simulink model "Einfachpendel_mit_Agent_19_09_22_17_13_35"  (R2022a)
settings: Solver=VariableStepAuto  StartTime=0.0  StopTime=Tf  RelTol=1e-3
PreLoadFcn:
  | init_Einfachpendel_mit_Agent
undefined symbols (not defined in the file or in its folder): d, Sample, theta0, X, x_lim, x_tar, Y, Z
libraries: sm_lib x15, nesl_utility x7, simulink x1, rllib x1
settings Model: Creator=ELSYS-PC3  LastModifiedBy=ts
settings SolverCC: AlgebraicLoopSolver=TrustRegion
settings DebuggingCC: UnconnectedInputMsg=warning  UnconnectedOutputMsg=warning  UnconnectedLineMsg=warning  SFMachineParentedDataDiag=warning  ArithmeticOperatorsInVariantConditions=warning
settings SFSimCC: SimUseLocalCustomCode=off  CustomCodeUndefinedFunction=UseInterfaceOnly
settings RTWCC: RTWUseLocalCustomCode=off  DLArmComputeVersion=19.05

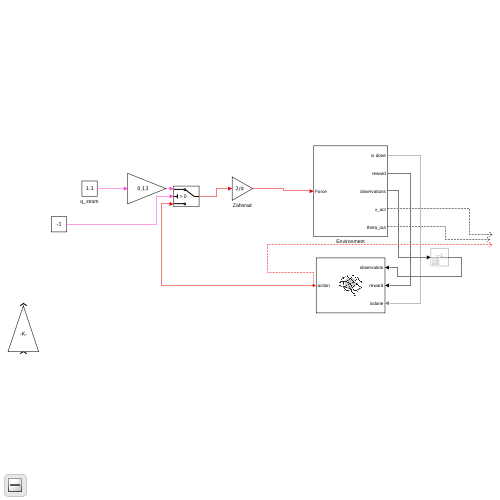
[thumbnail: Simulink's stored preview of the top-level diagram]
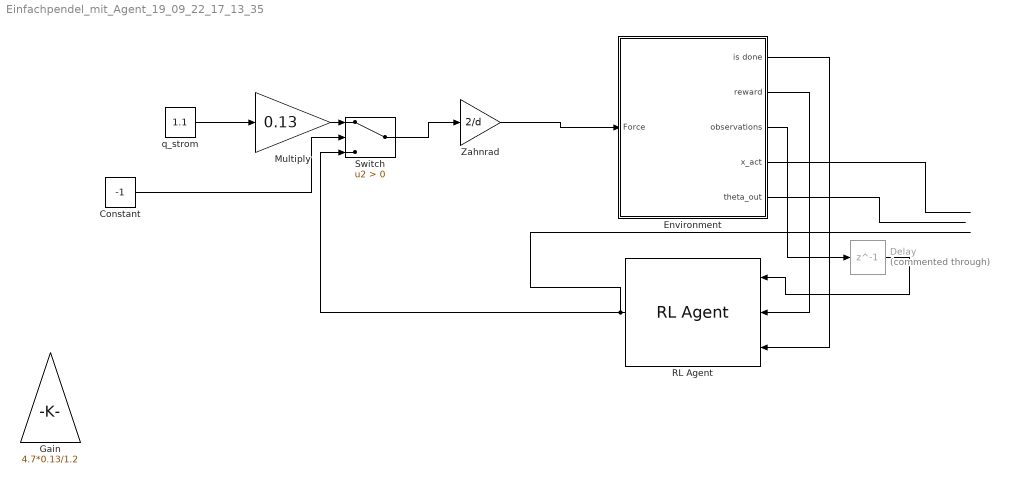
== system Einfachpendel_mit_Agent_19_09_22_17_13_35 ==
  Constant : Constant  Value=-1
  Delay : Delay  Commented=through  DelayLength=1
  Environment : Subsystem
  Gain : Gain  Gain=4.7*0.13/1.2
  Multiply : Gain  Gain=0.13
  RL Agent : rllib/RL Agent  Agent=bestagent  ExternalActionAsInput=off  ProvideLastAction=off  ProvideCumRwd=off  TreatAsDirectFeedthrough=on  UseStrictObservationDataTypes=off
  Switch : Switch  Criteria=u2 > Threshold  SaturateOnIntegerOverflow=off  InputSameDT=off
  Zahnrad : Gain  Gain=2/d
  q_strom : Constant  Value=1.1
  wires:
  Environment/1(is done) -> RL Agent/3
  Environment/2(reward) -> RL Agent/2
  Environment/4(x_act) -> ?
  Environment/5(theta_out) -> ?
  Environment/3(observations) -> Delay/1
  Delay/1 -> RL Agent/1
  Zahnrad/1 -> Environment/1(Force)
  q_strom/1 -> Multiply/1
  Switch/1 -> Zahnrad/1
  Constant/1 -> Switch/2
  Multiply/1 -> Switch/1
  RL Agent/1 -> Switch/3

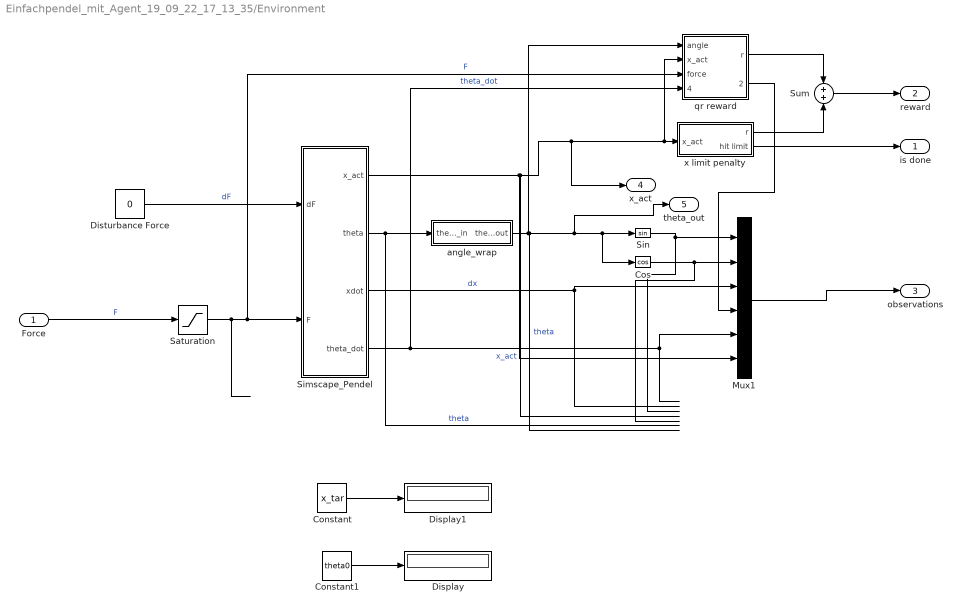
== system Einfachpendel_mit_Agent_19_09_22_17_13_35/Environment ==
  Force : Inport
  Constant : Constant  Value=x_tar
  Constant1 : Constant  Value=theta0
  Cos : Trigonometry  Operator=cos
  Display : Display
  Display1 : Display
  Disturbance Force : Constant  Value=0
  Mux1 : Mux  Inputs=6
  Saturation : Saturate  UpperLimit=140  LowerLimit=-140
  Simscape_Pendel : Subsystem
  Sin : Trigonometry
  Sum : Sum
  angle_wrap : Subsystem
  qr reward : Subsystem
  x limit penalty : Subsystem
  is done : Outport  VectorParamsAs1DForOutWhenUnconnected=off
  reward : Outport  Port=2  VectorParamsAs1DForOutWhenUnconnected=off
  observations : Outport  Port=3  VectorParamsAs1DForOutWhenUnconnected=off
  x_act : Outport  Port=4
  theta_out : Outport  Port=5
  wires:
  Mux1/1 -> observations/1
  Simscape_Pendel/3(xdot) -> Mux1/3  "dx"
  Simscape_Pendel/2("theta ") -> angle_wrap/1(theta_in)  "theta"
  Disturbance Force/1 -> Simscape_Pendel/1(dF)  "dF"
  angle_wrap/1(theta_out) -> theta_out/1, Cos/1, Sin/1, qr reward/1(angle)  "theta"
  Simscape_Pendel/4(theta_dot) -> qr reward/4(theta_dot), Mux1/5  "theta_dot"
  Sin/1 -> Mux1/1
  Cos/1 -> Mux1/2
  Sum/1 -> reward/1
  x limit penalty/2(hit limit) -> is done/1
  Saturation/1 -> Simscape_Pendel/2("F "), qr reward/3(force)  "F"
  qr reward/1(r) -> Sum/1
  x limit penalty/1(r) -> Sum/2
  Simscape_Pendel/1(x_act) -> Mux1/6, x_act/1, qr reward/2(x_act), x limit penalty/1(x_act)  "x_act"
  Force/1 -> Saturation/1  "F"
  Constant1/1 -> Display/1
  Constant/1 -> Display1/1
  qr reward/2(x_error) -> Mux1/4

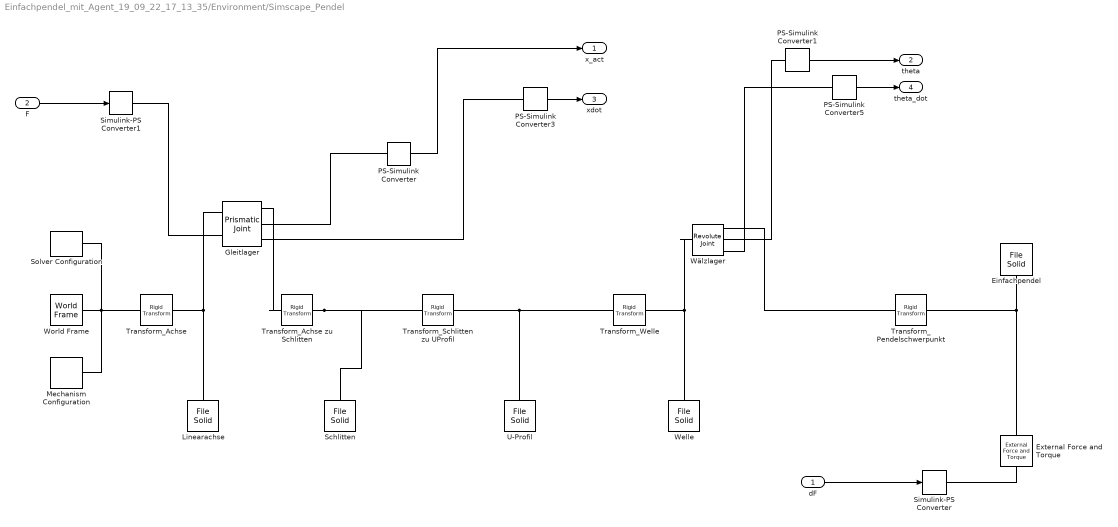
== system Einfachpendel_mit_Agent_19_09_22_17_13_35/Environment/Simscape_Pendel ==
  dF : Inport
  "F " : Inport  Port=2
  Einfachpendel : sm_lib/Body Elements/File Solid  ExtGeomFileName=/home/ts/Documents/2022_03_rosner_project2/Matlab/Pendel/V5_Einfachpendel_mit_Sollwertvorgabe/pendel2.stp  UnitType=FromFile  ExtGeomFileUnits=m  StepReaderType=OCC  ExportConvexHullGeometry=off  InertiaType=CalculateFromGeometry  Mass=1  MassUnits=kg  CenterOfMass=[0 0 0]  CenterOfMassUnits=m  MomentsOfInertia=[1 1 1]  MomentsOfInertiaUnits=kg*m^2  ProductsOfInertia=[0 0 0]  ProductsOfInertiaUnits=kg*m^2  BasedOnType=Density  Density=2710  DensityUnits=kg/m^3  DoExposeReferenceFrame=on  SerializedFrames=<Frames><Frame><Id>Frame1</Id><Value><Name>F1</Name><Origin><Source>CenterOfMassFrame</Source><FeatureName></FeatureName></Origin><PrimaryAxis><DefinedDirection>+Z</DefinedDirection><Source>ReferenceFrame</Source><SourceDirection>+Z</SourceDirection><FeatureName></FeatureName></PrimaryAxis><SecondaryAxis><DefinedDirection>+X</DefinedDirection><Source>ReferenceFrame</Source><SourceDirection>+X</SourceDirection><FeatureName></FeatureName></SecondaryAxis></Value></Frame></Frames>  GraphicType=FromGeometry  MarkerShape=Sphere  MarkerSize=10  GraphicVisPropType=SimpleVisualProperties  GraphicDiffuseColor=[1.0 0.2 0.4]  GraphicSpecularColor=[0.5 0.5 0.5 1.0]  GraphicAmbientColor=[0.15 0.15 0.15 1.0]  GraphicEmissiveColor=[0.0 0.0 0.0 1.0]  GraphicShininess=75  GraphicOpacity=1.0
  External Force and Torque : sm_lib/Forces and Torques/External Force and Torque  ForceResolutionFrame=AttachedFrame  EnableForceX=on  EnableForceY=off  EnableForceZ=off  EnableForce=off  TorqueResolutionFrame=AttachedFrame  EnableTorqueX=off  EnableTorqueY=off  EnableTorqueZ=off  EnableTorque=off
  Gleitlager : sm_lib/Joints/Prismatic Joint  JointMode=Normal  SenseConstraintForce=off  SenseConstraintForceX=off  SenseConstraintForceY=off  SenseConstraintForceZ=off  SenseConstraintTorque=off  SenseConstraintTorqueX=off  SenseConstraintTorqueY=off  SenseConstraintTorqueZ=off  SenseTotalForce=off  SenseTotalForceX=off  SenseTotalForceY=off  SenseTotalForceZ=off  SenseTotalTorque=off  SenseTotalTorqueX=off  SenseTotalTorqueY=off  SenseTotalTorqueZ=off  CompositeWrenchDir=FollowerOnBase  CompositeWrenchFrame=BaseFrame  EquilibriumPosition=0  EquilibriumPositionUnits=m  SpringStiffness=0  SpringStiffnessUnits=N/m  DampingCoefficient=46  DampingCoefficientUnits=N/(m/s)  TorqueActuationMode=InputTorque  MotionActuationMode=ComputedMotion  SensePosition=on  SenseVelocity=on  SenseAcceleration=off  SenseTorqueForce=off  SenseLowerLimitTorqueForce=off  SenseUpperLimitTorqueForce=off  LowerLimitSpecify=off  LowerLimitBound=-1  LowerLimitBoundUnits=m  LowerLimitStiffness=1e6  LowerLimitStiffnessUnits=N/m  LowerLimitDamping=1e3  LowerLimitDampingUnits=N/(m/s)  LowerLimitTransitionRegionWidth=1e-4  LowerLimitTransitionRegionWidthUnits=m  UpperLimitSpecify=off  UpperLimitBound=1  UpperLimitBoundUnits=m  UpperLimitStiffness=1e6  UpperLimitStiffnessUnits=N/m  UpperLimitDamping=1e3  UpperLimitDampingUnits=N/(m/s)  UpperLimitTransitionRegionWidth=1e-4  UpperLimitTransitionRegionWidthUnits=m  PositionTargetSpecify=on  PositionTargetPriority=High  PositionTargetValue=x_tar  PositionTargetValueUnits=m  VelocityTargetSpecify=on  VelocityTargetPriority=High  VelocityTargetValue=0  VelocityTargetValueUnits=m/s
  Linearachse : sm_lib/Body Elements/File Solid  ExtGeomFileName=/home/ts/Documents/2022_03_rosner_project2/Matlab/Pendel/V5_Einfachpendel_mit_Sollwertvorgabe/linearachse_asm.stp  UnitType=FromFile  ExtGeomFileUnits=m  StepReaderType=OCC  ExportConvexHullGeometry=off  InertiaType=CalculateFromGeometry  Mass=1  MassUnits=kg  CenterOfMass=[0 0 0]  CenterOfMassUnits=m  MomentsOfInertia=[1 1 1]  MomentsOfInertiaUnits=kg*m^2  ProductsOfInertia=[0 0 0]  ProductsOfInertiaUnits=kg*m^2  BasedOnType=Density  Density=3000  DensityUnits=kg/m^3  DoExposeReferenceFrame=on  SerializedFrames=<Frames/>  GraphicType=FromGeometry  MarkerShape=Sphere  MarkerSize=10  GraphicVisPropType=SimpleVisualProperties  GraphicDiffuseColor=[0.4 0.4 0.4]  GraphicSpecularColor=[0.5 0.5 0.5 1.0]  GraphicAmbientColor=[0.15 0.15 0.15 1.0]  GraphicEmissiveColor=[0.0 0.0 0.0 1.0]  GraphicShininess=75  GraphicOpacity=1.0
  Mechanism Configuration : sm_lib/Utilities/Mechanism Configuration  UniformGravity=Constant  GravityVector=[0 0 -9.80665]  GravityUnits=m/s^2  LinearizationDelta=0.001  JointModeTransitionNonlinearIterations=2
  PS-Simulink Converter{,1,3,5} (4 alike) : nesl_utility/PS-Simulink Converter  PhysicalDomain=network_engine_domain  SubClassName=ps_output  LeftPortType=input  RightPortType=output  PseudoPeriodic=off  Frequencies=[]  VectorFormat=1-D array  Unit=1  AffineConversion=off
      settings: SourceProductBaseCode=SS,PW,VE
  "Schlitten " : sm_lib/Body Elements/File Solid  ExtGeomFileName=/home/ts/Documents/2022_03_rosner_project2/Matlab/Pendel/V5_Einfachpendel_mit_Sollwertvorgabe/schlittenegc.stp  UnitType=FromFile  ExtGeomFileUnits=m  StepReaderType=OCC  ExportConvexHullGeometry=off  InertiaType=CalculateFromGeometry  Mass=1  MassUnits=kg  CenterOfMass=[0 0 0]  CenterOfMassUnits=m  MomentsOfInertia=[1 1 1]  MomentsOfInertiaUnits=kg*m^2  ProductsOfInertia=[0 0 0]  ProductsOfInertiaUnits=kg*m^2  BasedOnType=Density  Density=3000  DensityUnits=kg/m^3  DoExposeReferenceFrame=on  SerializedFrames=<Frames/>  GraphicType=FromGeometry  MarkerShape=Sphere  MarkerSize=10  GraphicVisPropType=SimpleVisualProperties  GraphicDiffuseColor=[0.5 0.5 0.5]  GraphicSpecularColor=[0.5 0.5 0.5 1.0]  GraphicAmbientColor=[0.15 0.15 0.15 1.0]  GraphicEmissiveColor=[0.0 0.0 0.0 1.0]  GraphicShininess=75  GraphicOpacity=1.0
  Simulink-PS Converter : nesl_utility/Simulink-PS Converter  PhysicalDomain=network_engine_domain  SubClassName=ps_input  LeftPortType=input  RightPortType=output  PseudoPeriodic=off  Frequencies=[]  NoiseDistribution=none  NoiseParameters=[]  Unit=1  AffineConversion=off  FilteringAndDerivatives=zero  SimscapeFilterOrder=1  InputFilterTimeConstant=0.001  UdotUserProvided=1
      settings: SourceProductBaseCode=SS,PW,VE
  Simulink-PS Converter1 : nesl_utility/Simulink-PS Converter  PhysicalDomain=network_engine_domain  SubClassName=ps_input  LeftPortType=input  RightPortType=output  PseudoPeriodic=off  Frequencies=[]  NoiseDistribution=none  NoiseParameters=[]  Unit=N  AffineConversion=off  FilteringAndDerivatives=zero  SimscapeFilterOrder=1  InputFilterTimeConstant=0.001  UdotUserProvided=1
      settings: SourceProductBaseCode=SS,PW,VE
  Solver Configuration : nesl_utility/Solver Configuration  PhysicalDomain=network_engine_domain  SubClassName=solver  LeftPortType=input  RightPortType=generic  Tones=[]  Harmonics=[]  SimulateNoise=off  Profile=off  UseLocalSampling=off  EnableSwitchedLinearOptims=on  FrequencyDomain=off  UseCCode=off  RelTol=0.001  AbsTol=1e-06  MinStep=1e-09  ToWorkspace=off  RevertToSquareIcSolve=off  NumHomotopyIterations=100  PhasorMode=off  PhasorModeNumHarmonics=1  IndexReductionMethod=DerivativeReplacement  DoDC=off  ResidualTolerance=1e-09  UseLocalSolver=off  LocalSolverChoice=NE_BACKWARD_EULER_ADVANCER  LocalSolverSampleTime=0.001  DoFixedCost=off  MaxNonlinIter=3  MaxModeIter=2  ComputeImpulses=off  ImpulseIterations=2  LinearAlgebra=Sparse  LinearAlgebraNumThread=0  EquationFormulation=NE_TIME_EF  DelaysMemoryBudget=1024  AutomaticFiltering=on  FilteringTimeConstant=0.001  PartitionStorageMethod=AS_NEEDED  PartitionMemoryBudget=1024  PartitionMethod=FAST
      settings: SourceProductBaseCode=SS,PW,VE
  Transform_Achse : sm_lib/Frames and Transforms/Rigid Transform  TranslationMethod=None  TranslationStandardOffset=0  TranslationLengthUnit=m  TranslationStandardAxis=+Z  TranslationCartesianOffset=[0 0 0]  TranslationROffset=0  TranslationROffsetUnits=m  TranslationZOffset=0  TranslationZOffsetUnits=m  TranslationThetaOffset=0  TranslationThetaOffsetUnits=deg  RotationMethod=AlignedAxes  RotationAngleUnits=deg  RotationStandardAxis=+Z  RotationAngle=0.0  RotationArbitraryAxis=[0 0 1]  FollAlignAxisA=+Z  BaseAlignAxisA=+X  FollAlignAxisB=+X  BaseAlignAxisB=+Y  RotationSequenceAxes=FollowerAxes  RotationSequence=XYX  RotationSequenceAngles=[0 0 0]  RotationSequenceAnglesUnits=deg  RotationMatrix=[1 0 0; 0 1 0; 0 0 1]
  Transform_Achse zu Schlitten : sm_lib/Frames and Transforms/Rigid Transform  TranslationMethod=Cartesian  TranslationStandardOffset=10/2+30/2  TranslationLengthUnit=mm  TranslationStandardAxis=+Y  TranslationCartesianOffset=[-67/2 44.3 100/2]  TranslationROffset=0  TranslationROffsetUnits=m  TranslationZOffset=0  TranslationZOffsetUnits=m  TranslationThetaOffset=0  TranslationThetaOffsetUnits=deg  RotationMethod=None  RotationAngleUnits=deg  RotationStandardAxis=+Z  RotationAngle=0.0  RotationArbitraryAxis=[0 0 1]  FollAlignAxisA=+Z  BaseAlignAxisA=+X  FollAlignAxisB=+X  BaseAlignAxisB=+Y  RotationSequenceAxes=FollowerAxes  RotationSequence=XYX  RotationSequenceAngles=[0 0 0]  RotationSequenceAnglesUnits=deg  RotationMatrix=[1 0 0; 0 1 0; 0 0 1]
  Transform_Pendelschwerpunkt : sm_lib/Frames and Transforms/Rigid Transform  TranslationMethod=Cartesian  TranslationStandardOffset=195.8  TranslationLengthUnit=mm  TranslationStandardAxis=+Y  TranslationCartesianOffset=[0 -195.8 8]  TranslationROffset=0  TranslationROffsetUnits=m  TranslationZOffset=0  TranslationZOffsetUnits=m  TranslationThetaOffset=0  TranslationThetaOffsetUnits=deg  RotationMethod=AlignedAxes  RotationAngleUnits=deg  RotationStandardAxis=+Z  RotationAngle=0.0  RotationArbitraryAxis=[0 0 1]  FollAlignAxisA=+Z  BaseAlignAxisA=+Y  FollAlignAxisB=+X  BaseAlignAxisB=+X  RotationSequenceAxes=FollowerAxes  RotationSequence=XYX  RotationSequenceAngles=[0 0 0]  RotationSequenceAnglesUnits=deg  RotationMatrix=[1 0 0; 0 1 0; 0 0 1]
  Transform_Schlitten zu UProfil : sm_lib/Frames and Transforms/Rigid Transform  TranslationMethod=Cartesian  TranslationStandardOffset=10/2+30/2  TranslationLengthUnit=mm  TranslationStandardAxis=+Y  TranslationCartesianOffset=[-27.5 18.7 10 ]  TranslationROffset=0  TranslationROffsetUnits=m  TranslationZOffset=0  TranslationZOffsetUnits=m  TranslationThetaOffset=0  TranslationThetaOffsetUnits=deg  RotationMethod=AlignedAxes  RotationAngleUnits=deg  RotationStandardAxis=+Z  RotationAngle=0.0  RotationArbitraryAxis=[0 0 1]  FollAlignAxisA=+X  BaseAlignAxisA=-Z  FollAlignAxisB=+Y  BaseAlignAxisB=+X  RotationSequenceAxes=FollowerAxes  RotationSequence=XYX  RotationSequenceAngles=[0 0 0]  RotationSequenceAnglesUnits=deg  RotationMatrix=[1 0 0; 0 1 0; 0 0 1]
  Transform_Welle : sm_lib/Frames and Transforms/Rigid Transform  TranslationMethod=Cartesian  TranslationStandardOffset=10/2+30/2  TranslationLengthUnit=mm  TranslationStandardAxis=+Y  TranslationCartesianOffset=[60 130 -56 ]  TranslationROffset=0  TranslationROffsetUnits=m  TranslationZOffset=0  TranslationZOffsetUnits=m  TranslationThetaOffset=0  TranslationThetaOffsetUnits=deg  RotationMethod=AlignedAxes  RotationAngleUnits=deg  RotationStandardAxis=+Z  RotationAngle=0.0  RotationArbitraryAxis=[0 0 1]  FollAlignAxisA=+Y  BaseAlignAxisA=+Z  FollAlignAxisB=+X  BaseAlignAxisB=+X  RotationSequenceAxes=FollowerAxes  RotationSequence=XYX  RotationSequenceAngles=[0 0 0]  RotationSequenceAnglesUnits=deg  RotationMatrix=[1 0 0; 0 1 0; 0 0 1]
  U-Profil : sm_lib/Body Elements/File Solid  ExtGeomFileName=/home/ts/Documents/2022_03_rosner_project2/Matlab/Pendel/V5_Einfachpendel_mit_Sollwertvorgabe/u_profil_asm.stp  UnitType=FromFile  ExtGeomFileUnits=m  StepReaderType=OCC  ExportConvexHullGeometry=off  InertiaType=CalculateFromGeometry  Mass=1  MassUnits=kg  CenterOfMass=[0 0 0]  CenterOfMassUnits=m  MomentsOfInertia=[1 1 1]  MomentsOfInertiaUnits=kg*m^2  ProductsOfInertia=[0 0 0]  ProductsOfInertiaUnits=kg*m^2  BasedOnType=Density  Density=2710  DensityUnits=kg/m^3  DoExposeReferenceFrame=on  SerializedFrames=<Frames/>  GraphicType=FromGeometry  MarkerShape=Sphere  MarkerSize=10  GraphicVisPropType=SimpleVisualProperties  GraphicDiffuseColor=[0.2 1.0 0.4]  GraphicSpecularColor=[0.5 0.5 0.5 1.0]  GraphicAmbientColor=[0.15 0.15 0.15 1.0]  GraphicEmissiveColor=[0.0 0.0 0.0 1.0]  GraphicShininess=75  GraphicOpacity=1.0
  Welle : sm_lib/Body Elements/File Solid  ExtGeomFileName=/home/ts/Documents/2022_03_rosner_project2/Matlab/Pendel/V5_Einfachpendel_mit_Sollwertvorgabe/welle.stp  UnitType=FromFile  ExtGeomFileUnits=m  StepReaderType=OCC  ExportConvexHullGeometry=off  InertiaType=CalculateFromGeometry  Mass=1  MassUnits=kg  CenterOfMass=[0 0 0]  CenterOfMassUnits=m  MomentsOfInertia=[1 1 1]  MomentsOfInertiaUnits=kg*m^2  ProductsOfInertia=[0 0 0]  ProductsOfInertiaUnits=kg*m^2  BasedOnType=Density  Density=7800  DensityUnits=kg/m^3  DoExposeReferenceFrame=on  SerializedFrames=<Frames/>  GraphicType=FromGeometry  MarkerShape=Sphere  MarkerSize=10  GraphicVisPropType=SimpleVisualProperties  GraphicDiffuseColor=[0.5 0.5 0.5]  GraphicSpecularColor=[0.5 0.5 0.5 1.0]  GraphicAmbientColor=[0.15 0.15 0.15 1.0]  GraphicEmissiveColor=[0.0 0.0 0.0 1.0]  GraphicShininess=75  GraphicOpacity=1.0
  World Frame : sm_lib/Frames and Transforms/World Frame
  Wälzlager : sm_lib/Joints/Revolute Joint  JointMode=Normal  SenseConstraintForce=off  SenseConstraintForceX=off  SenseConstraintForceY=off  SenseConstraintForceZ=off  SenseConstraintTorque=off  SenseConstraintTorqueX=off  SenseConstraintTorqueY=off  SenseConstraintTorqueZ=off  SenseTotalForce=off  SenseTotalForceX=off  SenseTotalForceY=off  SenseTotalForceZ=off  SenseTotalTorque=off  SenseTotalTorqueX=off  SenseTotalTorqueY=off  SenseTotalTorqueZ=off  CompositeWrenchDir=FollowerOnBase  CompositeWrenchFrame=BaseFrame  EquilibriumPosition=0  EquilibriumPositionUnits=deg  SpringStiffness=0  SpringStiffnessUnits=N*m/deg  DampingCoefficient=0.008594  DampingCoefficientUnits=N*m/(rad/s)  TorqueActuationMode=NoTorque  MotionActuationMode=ComputedMotion  SensePosition=on  SenseVelocity=on  SenseAcceleration=off  SenseTorqueForce=off  SenseLowerLimitTorqueForce=off  SenseUpperLimitTorqueForce=off  LowerLimitSpecify=off  LowerLimitBound=-90  LowerLimitBoundUnits=deg  LowerLimitStiffness=1e4  LowerLimitStiffnessUnits=N*m/deg  LowerLimitDamping=10  LowerLimitDampingUnits=N*m/(deg/s)  LowerLimitTransitionRegionWidth=0.1  LowerLimitTransitionRegionWidthUnits=deg  UpperLimitSpecify=off  UpperLimitBound=90  UpperLimitBoundUnits=deg  UpperLimitStiffness=1e4  UpperLimitStiffnessUnits=N*m/deg  UpperLimitDamping=10  UpperLimitDampingUnits=N*m/(deg/s)  UpperLimitTransitionRegionWidth=0.1  UpperLimitTransitionRegionWidthUnits=deg  PositionTargetSpecify=on  PositionTargetPriority=High  PositionTargetValue=theta0  PositionTargetValueUnits=rad  VelocityTargetSpecify=off  VelocityTargetPriority=High  VelocityTargetValue=0  VelocityTargetValueUnits=deg/s
  x_act : Outport  VectorParamsAs1DForOutWhenUnconnected=off
  "theta " : Outport  Port=2  VectorParamsAs1DForOutWhenUnconnected=off
  xdot : Outport  Port=3  VectorParamsAs1DForOutWhenUnconnected=off
  theta_dot : Outport  Port=4  VectorParamsAs1DForOutWhenUnconnected=off
  wires:
  PS-Simulink Converter5/1 -> theta_dot/1
  "F "/1 -> Simulink-PS Converter1/1
  PS-Simulink Converter1/1 -> "theta "/1
  dF/1 -> Simulink-PS Converter/1
  PS-Simulink Converter3/1 -> xdot/1
  PS-Simulink Converter/1 -> x_act/1
  connections:
  Transform_Achse/RConn1 -- Gleitlager/LConn1 -- Linearachse/RConn1
  External Force and Torque/RConn1 -- Transform_Pendelschwerpunkt/RConn1 -- Einfachpendel/LConn1
  Mechanism Configuration/RConn1 -- Transform_Achse/LConn1 -- World Frame/RConn1 -- Solver Configuration/RConn1
  Transform_Welle/RConn1 -- Welle/RConn1 -- Wälzlager/LConn1
  Transform_Achse zu Schlitten/RConn1 -- "Schlitten "/RConn1 -- Transform_Schlitten zu UProfil/LConn1
  Transform_Schlitten zu UProfil/RConn1 -- Transform_Welle/LConn1 -- U-Profil/RConn1
  Wälzlager/RConn3 -- PS-Simulink Converter5/LConn1
  Wälzlager/RConn2 -- PS-Simulink Converter1/LConn1
  Gleitlager/RConn2 -- PS-Simulink Converter/LConn1
  Simulink-PS Converter/RConn1 -- External Force and Torque/LConn1
  Transform_Achse zu Schlitten/LConn1 -- Gleitlager/RConn1
  Transform_Pendelschwerpunkt/LConn1 -- Wälzlager/RConn1
  PS-Simulink Converter3/LConn1 -- Gleitlager/RConn3
  Simulink-PS Converter1/RConn1 -- Gleitlager/LConn2

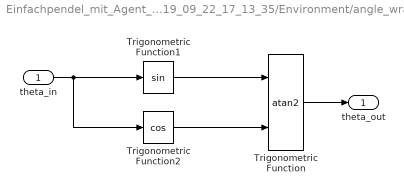
== system Einfachpendel_mit_Agent_19_09_22_17_13_35/Environment/angle_wrap ==
  theta_in : Inport
  Trigonometric Function : Trigonometry  Operator=atan2
  Trigonometric Function1 : Trigonometry
  Trigonometric Function2 : Trigonometry  Operator=cos
  theta_out : Outport  VectorParamsAs1DForOutWhenUnconnected=off
  wires:
  theta_in/1 -> Trigonometric Function2/1, Trigonometric Function1/1
  Trigonometric Function/1 -> theta_out/1
  Trigonometric Function1/1 -> Trigonometric Function/1
  Trigonometric Function2/1 -> Trigonometric Function/2

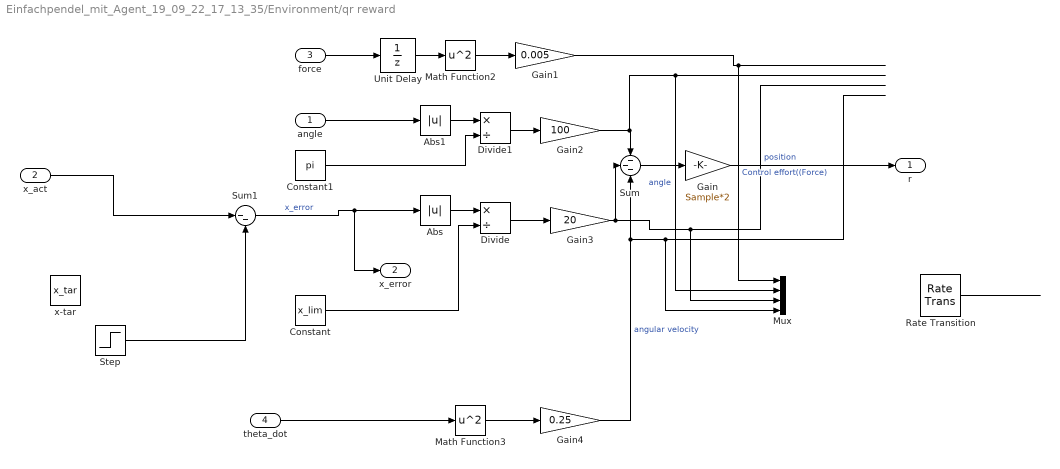
== system Einfachpendel_mit_Agent_19_09_22_17_13_35/Environment/qr reward ==
  angle : Inport
  x_act : Inport  Port=2
  force : Inport  Port=3
  theta_dot : Inport  Port=4
  Abs : Abs  SaturateOnIntegerOverflow=off
  Abs1 : Abs  SaturateOnIntegerOverflow=off
  Constant : Constant  Value=x_lim
  Constant1 : Constant  Value=pi
  Divide : Product  Inputs=*/
  Divide1 : Product  Inputs=*/
  Gain : Gain  Gain=Sample*2
  Gain1 : Gain  Gain=0.005
  Gain2 : Gain  Gain=100
  Gain3 : Gain  Gain=20
  Gain4 : Gain  Gain=0.25
  Math Function2 : Math  Operator=square  SignedPower=on
  Math Function3 : Math  Operator=square  SignedPower=on
  Mux : Mux
  Rate Transition : RateTransition  OutPortSampleTime=Sample
  Step : Step  Time=5  After=x_tar  SampleTime=0
  Sum : Sum  Inputs=---
  Sum1 : Sum  Inputs=|--
  Unit Delay : UnitDelay  SampleTime=-1  HasFrameUpgradeWarning=on
  x-tar : Constant  Value=x_tar
  r : Outport  VectorParamsAs1DForOutWhenUnconnected=off
  x_error : Outport  Port=2
  wires:
  angle/1 -> Abs1/1
  Gain3/1 -> Sum/2, Mux/3  "position"
  force/1 -> Unit Delay/1
  Gain1/1 -> Mux/1  "Control effort((Force)"
  Sum/1 -> Gain/1
  Unit Delay/1 -> Math Function2/1
  Gain4/1 -> Sum/3, Mux/4  "angular velocity"
  theta_dot/1 -> Math Function3/1
  Math Function2/1 -> Gain1/1
  Math Function3/1 -> Gain4/1
  Abs/1 -> Divide/1
  Divide/1 -> Gain3/1
  Constant/1 -> Divide/2
  Abs1/1 -> Divide1/1
  Divide1/1 -> Gain2/1
  Gain2/1 -> Mux/2, Sum/1  "angle"
  Constant1/1 -> Divide1/2
  Gain/1 -> r/1
  Rate Transition/1 -> ?
  x_act/1 -> Sum1/1
  Sum1/1 -> x_error/1, Abs/1  "x_error"
  Step/1 -> Sum1/2

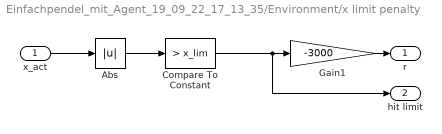
== system Einfachpendel_mit_Agent_19_09_22_17_13_35/Environment/x limit penalty ==
  x_act : Inport
  Abs : Abs  SaturateOnIntegerOverflow=off
  Compare To Constant : simulink/Logic and Bit Operations/Compare To Constant  relop=>  const=x_lim  OutDataTypeStr=boolean
  Gain1 : Gain  Gain=-3000
  r : Outport  VectorParamsAs1DForOutWhenUnconnected=off
  hit limit : Outport  Port=2  VectorParamsAs1DForOutWhenUnconnected=off
  wires:
  Gain1/1 -> r/1
  x_act/1 -> Abs/1
  Abs/1 -> Compare To Constant/1
  Compare To Constant/1 -> hit limit/1, Gain1/1
